simulink model "FOC_Motor_Tuning"  (R2025b)
settings: Solver=VariableStepAuto  StartTime=0.0  StopTime=8  RelTol=1e-3
values from neighbouring files (symbols this model uses):
  adc : value not decoded    [FoCFpgaData.sldd]
  dataRange = 800.0    [FoCFpgaData.sldd]
  encoder = 0.0    [FoCFpgaData.sldd]
  inverter = 24.0    [FoCFpgaData.sldd]
  paramAdcAmperePerCount : value not decoded    [FoCFpgaData.sldd]
  paramAdcCalibrationSamples = 16.0    [FoCFpgaData.sldd]
  paramAdcCountAtZeroAmpere : value not decoded    [FoCFpgaData.sldd]
  paramAdcEnablecalibration = 1.0    [FoCFpgaData.sldd]
  paramCurrentControlSatVoltage = 13.856406460551021    [FoCFpgaData.sldd]
  paramEncoderCalibrationDuration = 0.2    [FoCFpgaData.sldd]
  paramEncoderCalibrationMaxError = 0.0012566370614359172    [FoCFpgaData.sldd]
  paramEncoderCalibrationVoltage = 2.0    [FoCFpgaData.sldd]
  paramEncoderRotorPositionAtZeroCount = 0.0    [FoCFpgaData.sldd]
  paramOpenLoopVelocityAcceleration = 40.0    [FoCFpgaData.sldd]
  paramOpenLoopVelocityToVoltsBias = 0.4    [FoCFpgaData.sldd]
  paramOpenLoopVelocityToVoltsScalar = 0.04    [FoCFpgaData.sldd]
  paramOverCurrentDuration = 0.05    [FoCFpgaData.sldd]
  paramOverCurrentEnable = 0.0    [FoCFpgaData.sldd]
  paramOverCurrentLimit = 10.45    [FoCFpgaData.sldd]
  paramPwmCompareAtZeroVolt = 500.0    [FoCFpgaData.sldd]
  paramPwmCompareMax = 1000.0    [FoCFpgaData.sldd]
  paramPwmComparePerVolt = 41.666666666666664    [FoCFpgaData.sldd]
  paramVelocityControlSatCurrent = 3.5    [FoCFpgaData.sldd]
  PI_params = 0.00048000000000000007    [FoCFpgaData.sldd]
  pmsm : value not decoded    [FoCFpgaData.sldd]
  pwm = 2.0E-8    [FoCFpgaData.sldd]
  sampleTime = 4.0E-5    [FoCFpgaData.sldd]
libraries: fl_lib x12, nesl_utility x12, mcbeeMathTransformLib x8, simulink x4, slpidlib x4, ee_lib x4, mcbpositiondecoderlib x3, mcbcontrolslib x3, mcbplantlib x1, autolibpmsmexterior x1, eeGeneralControl x1, SignalEditorBlockLib x1
(part 3 of 3)

== system FOC_Motor_Tuning/FOC Control/Controller_Algorithm_Local/Algorithm_С/Open_Loop_Velocity_Control/Open_Loop_Velocity_Control/Inverse_Park_Transform ==
  note: Inverse Park Transform
  note: Converts orthogonal rotating reference frame (dq) to two-phase orthogonal stationary reference frame (alpha, beta)
  D : Inport
  Q : Inport  Port=2
  Sin_Coefficient : Inport  Port=3
  Cos_Coefficient : Inport  Port=4
  Add1 : Sum  Inputs=+-  OutDataTypeStr=Inherit: Same as first input
  Add2 : Sum  OutDataTypeStr=Inherit: Same as first input
  Cos_Coefficient1 : InportShadow  Port=4
  Product{1..4} (4 alike) : Product  RndMeth=Simplest
  Sin_Coefficient1 : InportShadow  Port=3
  Alpha : Outport  VectorParamsAs1DForOutWhenUnconnected=off
  Beta : Outport  Port=2  VectorParamsAs1DForOutWhenUnconnected=off
  wires:
  Add2/1 -> Beta/1
  Add1/1 -> Alpha/1
  Product3/1 -> Add2/1
  Product4/1 -> Add2/2
  Product1/1 -> Add1/1
  Product2/1 -> Add1/2
  Cos_Coefficient1/1 -> Product4/2
  Sin_Coefficient/1 -> Product2/2
  D/1 -> Product3/1, Product1/1
  Q/1 -> Product2/1, Product4/1
  Sin_Coefficient1/1 -> Product3/2
  Cos_Coefficient/1 -> Product1/2

== system FOC_Motor_Tuning/FOC Control/Controller_Algorithm_Local/Algorithm_С/Open_Loop_Velocity_Control/Open_Loop_Velocity_Control/Ramp_Velocity ==
  note: Ramp Velocity
  Velocity_Command : Inport
  Delay : Delay  DelayLength=1
  Gain : Gain  Gain=sampleTime.OpenLoopVelocityControl
      settings: AttributesFormatString=------------------------------\nGain = %<Gain>
  Number_Of_Pole_Pairs : Gain  Gain=pmsm.p
      settings: AttributesFormatString=------------------------------------\nGain = %<Gain>
  Set_Acceleration : Subsystem
  Sum : Sum  Inputs=++|  SaturateOnIntegerOverflow=on
  Rotor_Velocity : Outport  VectorParamsAs1DForOutWhenUnconnected=off
  Electrical_Velocity : Outport  Port=2  VectorParamsAs1DForOutWhenUnconnected=off
  wires:
  Number_Of_Pole_Pairs/1 -> Electrical_Velocity/1
  Set_Acceleration/1(A) -> Gain/1
  Velocity_Command/1 -> Set_Acceleration/1(V_Target)
  Gain/1 -> Sum/1
  Delay/1 -> Set_Acceleration/2(V_Current), Sum/2, Number_Of_Pole_Pairs/1, Rotor_Velocity/1
  Sum/1 -> Delay/1

== system FOC_Motor_Tuning/FOC Control/Controller_Algorithm_Local/Algorithm_С/Open_Loop_Velocity_Control/Open_Loop_Velocity_Control/Rotor_Velocity_To_Volts ==
  note: Rotor Velocity To Volts
  RV : Inport
  Abs : Abs  SaturateOnIntegerOverflow=off
  Add : Sum  OutDataTypeStr=Inherit: Same as first input
  Frequency_To_Voltage : Gain  Gain=paramOpenLoopVelocityToVoltsScalar
      settings: AttributesFormatString=--------------------------------\n%<Gain>
  Voltage_Bias : Constant  Value=paramOpenLoopVelocityToVoltsBias  OutDataTypeStr=Inherit: Inherit via back propagation  SampleTime=-1
  V : Outport  VectorParamsAs1DForOutWhenUnconnected=off
  wires:
  RV/1 -> Abs/1
  Abs/1 -> Frequency_To_Voltage/1
  Frequency_To_Voltage/1 -> Add/2
  Add/1 -> V/1
  Voltage_Bias/1 -> Add/1

== system FOC_Motor_Tuning/FOC Control/Controller_Algorithm_Local/Algorithm_HDL/FOC_Velocity_Encoder/FOC_Current_Control/FOC_Current_Control_Fixdt/DQ_Current_Control ==
  note: DQ Current Control
  Reset : Inport
  Q_Command : Inport  Port=2  SampleTime=sampleTime.CurrentControl
  D_Current : Inport  Port=3
  Q_Current : Inport  Port=4
  D_Command : Constant  Value=0  OutDataTypeStr=fixdt(1,16,0)  SampleTime=-1
  D_Control : slpidlib/PID Controller  Controller=PI  Form=Parallel  TimeDomain=Discrete-time  UseExternalTs=off  SampleTime=-1  IntegratorMethod=Forward Euler  FilterMethod=Forward Euler  ControllerParametersSource=external  P=1  I=1  UseKiTs=on  D=0  UseExternalDerivativeSource=off  N=100  UseFilter=on  TunerSelectOption=Transfer Function Based (PID Tuner App)  InitialConditionSource=internal  InitialConditionForIntegrator=0  InitialConditionForFilter=0  DifferentiatorICPrevScaledInput=0  ExternalReset=level  TrackingMode=off  Kt=1  LimitOutput=on  SatLimitsSource=internal  UpperSaturationLimit=paramCurrentControlSatVoltage  LowerSaturationLimit=-paramCurrentControlSatVoltage  LinearizeAsGain=on  AntiWindupMode=clamping  Kb=1  LimitIntegrator=off  UpperIntegratorSaturationLimit=inf  LowerIntegratorSaturationLimit=-inf  RndMeth=Simplest  POutMin=[]  POutMax=[]  IOutMin=[]  IOutMax=[]  DOutMin=[]  DOutMax=[]  NOutMin=[]  NOutMax=[]  SumOutMin=[]  SumOutMax=[]  SaturationOutDataTypeStr=Inherit: Inherit via back propagation  SaturationOutMin=[]  SaturationOutMax=[]  PParamMin=[]  PParamMax=[]  IParamMin=[]  IParamMax=[]  DParamMin=[]  DParamMax=[]  NParamMin=[]  NParamMax=[]  KbParamMin=[]  KbParamMax=[]  KtParamMin=[]  KtParamMax=[]  KbOutMin=[]  KbOutMax=[]  KtOutMin=[]  KtOutMax=[]  IntegratorOutMin=[]  IntegratorOutMax=[]  FilterOutMin=[]  FilterOutMax=[]  SumI1OutMin=[]  SumI1OutMax=[]  SumI2OutMin=[]  SumI2OutMax=[]  SumI3OutMin=[]  SumI3OutMax=[]  SumI4OutMin=[]  SumI4OutMax=[]  SumDOutMin=[]  SumDOutMax=[]  DifferentiatorOutMin=[]  DifferentiatorOutMax=[]  FilterDiffOutCoefMin=[]  FilterDiffOutCoefMax=[]  ReciprocalOutMin=[]  ReciprocalOutMax=[]  SumDenOutMin=[]  SumDenOutMax=[]  SumNumOutMin=[]  SumNumOutMax=[]  DivideOutMin=[]  DivideOutMax=[]  UdiffTsProdOutMin=[]  UdiffTsProdOutMax=[]  NTsProdOutMin=[]  NTsProdOutMax=[]  UintegralTsProdOutMin=[]  UintegralTsProdOutMax=[]  UngainTsProdOutMin=[]  UngainTsProdOutMax=[]  ClampingZeroOutDataTypeStr=Inherit: Inherit via back propagation  ClampingZeroOutMin=[]  ClampingZeroOutMax=[]  FilterDenConstantOutDataTypeStr=Inherit: Inherit via back propagation  FilterDenConstantOutMin=[]  FilterDenConstantOutMax=[]  PCopyOutDataTypeStr=Inherit: Inherit via back propagation  PCopyOutMin=[]  PCopyOutMax=[]  NCopyOutDataTypeStr=Inherit: Inherit via back propagation  NCopyOutMin=[]  NCopyOutMax=[]  IntegratorContinuousStateAttributes=''  IntegratorStateMustResolveToSignalObject=off  IntegratorRTWStateStorageClass=Auto  FilterContinuousStateAttributes=''  FilterStateMustResolveToSignalObject=off  FilterRTWStateStorageClass=Auto  ParallelPVariant=ExternalParameters  IdealPVariant=Disabled  IVariant=ExternalParameters  DVariant=Disabled  IntegratorVariant=Discrete  SatVariant=Enabled  AWVariant=DiscClampingParallel  PCopyVariant=Disabled  TRVariant=Disabled  FdbkBlocksVariant=Forward  IdealPFdbkVariant=Disabled  SatFdbkVariant=Disabled  DerivativeFilterVariant=Disabled  NVariant=Disabled  NCopyVariant=Disabled_SignalSpec  FilterICVariant=Disabled  IntegratorICVariant=InternalICs  ExternalResetVariant=ExternalReset  TRSumVariant=Passthrough  SumFdbkVariant=Disabled  SumVariant=Sum_PI  TsampFilterVariant=InternalTs  TsampNgainVariant=Passthrough  TsampIntegralVariant=Disabled_SignalSpec  ExternalSaturationOutDataTypeStr=Inherit: Same as second input  DerivativeSourceVariant=Disabled  PreIntVariant=InternalPreInt
      settings: LibrarySourceBlock=mcblib/Controls/Controllers/PI Controller
  Data_Type_Convert : DataTypeConversion  OutDataTypeStr=fixdt(1,16,11)  RndMeth=Simplest  SaturateOnIntegerOverflow=off
  Data_Type_Convert1 : DataTypeConversion  OutDataTypeStr=fixdt(1,16,11)  RndMeth=Simplest  SaturateOnIntegerOverflow=off
  Error : Sum  Inputs=+-  OutDataTypeStr=fixdt(1,32,24)
  Error1 : Sum  Inputs=+-  OutDataTypeStr=fixdt(1,32,24)
  Integral_Gain : Constant  Value=PI_params.Ki_i  OutDataTypeStr=fixdt(1,16,3)  SampleTime=-1
  Integral_Gain1 : Constant  Value=PI_params.Kp_i  OutDataTypeStr=fixdt(1,16,3)  SampleTime=-1
  Product : Product  OutDataTypeStr=fixdt(1,16,15)
  Q_Control : slpidlib/PID Controller  Controller=PI  Form=Parallel  TimeDomain=Discrete-time  UseExternalTs=off  SampleTime=-1  IntegratorMethod=Forward Euler  FilterMethod=Forward Euler  ControllerParametersSource=external  P=1  I=1  UseKiTs=on  D=0  UseExternalDerivativeSource=off  N=100  UseFilter=on  TunerSelectOption=Transfer Function Based (PID Tuner App)  InitialConditionSource=internal  InitialConditionForIntegrator=0  InitialConditionForFilter=0  DifferentiatorICPrevScaledInput=0  ExternalReset=level  TrackingMode=off  Kt=1  LimitOutput=on  SatLimitsSource=internal  UpperSaturationLimit=paramCurrentControlSatVoltage  LowerSaturationLimit=-paramCurrentControlSatVoltage  LinearizeAsGain=on  AntiWindupMode=clamping  Kb=1  LimitIntegrator=off  UpperIntegratorSaturationLimit=inf  LowerIntegratorSaturationLimit=-inf  RndMeth=Simplest  POutMin=[]  POutMax=[]  IOutMin=[]  IOutMax=[]  DOutMin=[]  DOutMax=[]  NOutMin=[]  NOutMax=[]  SumOutMin=[]  SumOutMax=[]  SaturationOutDataTypeStr=Inherit: Inherit via back propagation  SaturationOutMin=[]  SaturationOutMax=[]  PParamMin=[]  PParamMax=[]  IParamMin=[]  IParamMax=[]  DParamMin=[]  DParamMax=[]  NParamMin=[]  NParamMax=[]  KbParamMin=[]  KbParamMax=[]  KtParamMin=[]  KtParamMax=[]  KbOutMin=[]  KbOutMax=[]  KtOutMin=[]  KtOutMax=[]  IntegratorOutMin=[]  IntegratorOutMax=[]  FilterOutMin=[]  FilterOutMax=[]  SumI1OutMin=[]  SumI1OutMax=[]  SumI2OutMin=[]  SumI2OutMax=[]  SumI3OutMin=[]  SumI3OutMax=[]  SumI4OutMin=[]  SumI4OutMax=[]  SumDOutMin=[]  SumDOutMax=[]  DifferentiatorOutMin=[]  DifferentiatorOutMax=[]  FilterDiffOutCoefMin=[]  FilterDiffOutCoefMax=[]  ReciprocalOutMin=[]  ReciprocalOutMax=[]  SumDenOutMin=[]  SumDenOutMax=[]  SumNumOutMin=[]  SumNumOutMax=[]  DivideOutMin=[]  DivideOutMax=[]  UdiffTsProdOutMin=[]  UdiffTsProdOutMax=[]  NTsProdOutMin=[]  NTsProdOutMax=[]  UintegralTsProdOutMin=[]  UintegralTsProdOutMax=[]  UngainTsProdOutMin=[]  UngainTsProdOutMax=[]  ClampingZeroOutDataTypeStr=Inherit: Inherit via back propagation  ClampingZeroOutMin=[]  ClampingZeroOutMax=[]  FilterDenConstantOutDataTypeStr=Inherit: Inherit via back propagation  FilterDenConstantOutMin=[]  FilterDenConstantOutMax=[]  PCopyOutDataTypeStr=Inherit: Inherit via back propagation  PCopyOutMin=[]  PCopyOutMax=[]  NCopyOutDataTypeStr=Inherit: Inherit via back propagation  NCopyOutMin=[]  NCopyOutMax=[]  IntegratorContinuousStateAttributes=''  IntegratorStateMustResolveToSignalObject=off  IntegratorRTWStateStorageClass=Auto  FilterContinuousStateAttributes=''  FilterStateMustResolveToSignalObject=off  FilterRTWStateStorageClass=Auto  ParallelPVariant=ExternalParameters  IdealPVariant=Disabled  IVariant=ExternalParameters  DVariant=Disabled  IntegratorVariant=Discrete  SatVariant=Enabled  AWVariant=DiscClampingParallel  PCopyVariant=Disabled  TRVariant=Disabled  FdbkBlocksVariant=Forward  IdealPFdbkVariant=Disabled  SatFdbkVariant=Disabled  DerivativeFilterVariant=Disabled  NVariant=Disabled  NCopyVariant=Disabled_SignalSpec  FilterICVariant=Disabled  IntegratorICVariant=InternalICs  ExternalResetVariant=ExternalReset  TRSumVariant=Passthrough  SumFdbkVariant=Disabled  SumVariant=Sum_PI  TsampFilterVariant=InternalTs  TsampNgainVariant=Passthrough  TsampIntegralVariant=Disabled_SignalSpec  ExternalSaturationOutDataTypeStr=Inherit: Same as second input  DerivativeSourceVariant=Disabled  PreIntVariant=InternalPreInt
      settings: LibrarySourceBlock=mcblib/Controls/Controllers/PI Controller
  Reset1 : InportShadow
  Sample_Time : Constant  Value=sampleTime.CurrentControl  OutDataTypeStr=fixdt(1,16,27)  SampleTime=-1
  D_Voltage : Outport  VectorParamsAs1DForOutWhenUnconnected=off
  Q_Voltage : Outport  Port=2  VectorParamsAs1DForOutWhenUnconnected=off
  wires:
  Data_Type_Convert1/1 -> Q_Voltage/1
  D_Control/1 -> Data_Type_Convert/1
  D_Command/1 -> Error/1  "Id_Ref"
  Q_Command/1 -> Error1/1  "Iq_Ref"
  Q_Current/1 -> Error1/2  "Iq_Fb"
  D_Current/1 -> Error/2  "Id_Fb"
  Reset/1 -> D_Control/4
  Reset1/1 -> Q_Control/4
  Error/1 -> D_Control/1  "currentControlError"
  Product/1 -> Q_Control/3, D_Control/3
  Sample_Time/1 -> Product/2
  Integral_Gain/1 -> Product/1
  Integral_Gain1/1 -> Q_Control/2, D_Control/2
  Data_Type_Convert/1 -> D_Voltage/1
  Q_Control/1 -> Data_Type_Convert1/1
  Error1/1 -> Q_Control/1  "currentControlError"

== system FOC_Motor_Tuning/FOC Control/Controller_Algorithm_Local/Algorithm_HDL/FOC_Velocity_Encoder/FOC_Current_Control/FOC_Current_Control_Fixdt/Sine_Cosine ==
  note: Sine Cosine Fixed Point LUT
  P : Inport
  Normalize_Position : Gain  Gain=1/(2*pi)  ParamDataTypeStr=fixdt(1,16,17)  OutMin=0  OutMax=1  OutDataTypeStr=fixdt(1,32,30)
      settings: AttributesFormatString=|
      | ------------------------------
      | Gain = %<Gain>
  Sine_Cosine_LUT : simulink/Lookup Tables/Sine  Formula=sin(2*pi*u) and cos(2*pi*u)  NumDataPoints=(2^5)+1  OutputWordLength=16  InternalRulePriority=Speed
  Sin : Outport  VectorParamsAs1DForOutWhenUnconnected=off
  Cos : Outport  Port=2  VectorParamsAs1DForOutWhenUnconnected=off
  wires:
  Sine_Cosine_LUT/2 -> Cos/1
  Sine_Cosine_LUT/1 -> Sin/1
  Normalize_Position/1 -> Sine_Cosine_LUT/1
  P/1 -> Normalize_Position/1  "position"

== system FOC_Motor_Tuning/FOC Control/Controller_Algorithm_Local/Algorithm_HDL/FOC_Velocity_Encoder/FOC_Current_Control/FOC_Current_Control_Single/FOC_Current_Control ==
  note: FOC Current Control
  Reset : Inport  SampleTime=sampleTime.CurrentControl
  Current_Command : Inport  Port=2  OutMin=dataRange.PhaseCurrent.Min  OutMax=dataRange.PhaseCurrent.Max  SampleTime=sampleTime.CurrentControl
  Phase_Current : Inport  Port=3  OutMin=dataRange.PhaseCurrent.Min  OutMax=dataRange.PhaseCurrent.Max  SampleTime=sampleTime.CurrentControl
  Electrical_Position : Inport  Port=4  OutMin=0  OutMax=2*pi  SampleTime=sampleTime.CurrentControl
  Clarke Transform : mcbeeMathTransformLib/Clarke Transform  VariantControl=Variant2  PowerInvariant=off  UseWithEmbedded=on  PhaseInput=Two inputs
      settings: LibrarySourceBlock=mcbcontrolslib/Clarke Transform
  DQ_Current_Control : Subsystem
  Demux : Demux  Outputs=2
  Inverse Clarke Transform : mcbeeMathTransformLib/Inverse Clarke Transform  PowerInvariant=off  UseWithEmbedded=on  PhaseInput=Two inputs
      settings: LibrarySourceBlock=mcbcontrolslib/Inverse Clarke Transform
  Inverse Park Transform : mcbeeMathTransformLib/Park to Clarke Angle Transform  AxisAlignment=D-axis  UseWithEmbedded=on  PhaseInput=Two inputs  ThetaInput=Sine and Cosine electrical position  AngleInput=Per-unit  N_points=1024
      settings: LibrarySourceBlock=mcbcontrolslib/Inverse Park Transform
  Mux : Mux  Inputs=3
  PWM Reference Generator : mcbcontrolslib/PWM Reference Generator  inSignal=Vabc  modType=SVM: space vector modulation
      settings: LibrarySourceBlock=mcbhdllib/Controls/Math Transforms/PWM Reference Generator
  Park Transform : mcbeeMathTransformLib/Clarke to Park Angle Transform  AxisAlignment=D-axis  UseWithEmbedded=on  PhaseInput=Two inputs  ThetaInput=Sine and Cosine electrical position  AngleInput=Per-unit  N_points=1024
      settings: LibrarySourceBlock=mcbcontrolslib/Park Transform
  Sat : Saturate  UpperLimit=dataRange.PhaseVoltage.Max  LowerLimit=dataRange.PhaseVoltage.Min  OutDataTypeStr=Inherit: Inherit via back propagation
      settings: AttributesFormatString=-----------------\nLower = %<LowerLimit>\nUpper = %<UpperLimit>
  Trigonometric Function : Trigonometry  Operator=sincos
  Phase_Voltage : Outport  SampleTime=sampleTime.CurrentControl  VectorParamsAs1DForOutWhenUnconnected=off
  wires:
  Trigonometric Function/1 -> Inverse Park Transform/3, Park Transform/3  "sinCoefficient"
  Trigonometric Function/2 -> Inverse Park Transform/4, Park Transform/4  "cosCoefficient"
  Electrical_Position/1 -> Trigonometric Function/1
  Clarke Transform/1 -> Park Transform/1  "alphaCurrent"
  Clarke Transform/2 -> Park Transform/2  "betaCurrent"
  Inverse Park Transform/1 -> Inverse Clarke Transform/1  "alphaVoltage"
  Inverse Park Transform/2 -> Inverse Clarke Transform/2  "betaVoltage"
  Park Transform/1 -> DQ_Current_Control/3(D_Current)  "dCurrent"
  Park Transform/2 -> DQ_Current_Control/4(Q_Current)  "qCurrent"
  Current_Command/1 -> DQ_Current_Control/2(Q_Command)
  DQ_Current_Control/1(D_Voltage) -> Inverse Park Transform/1  "dVoltage"
  DQ_Current_Control/2(Q_Voltage) -> Inverse Park Transform/2  "qVoltage"
  Mux/1 -> Sat/1  "svmVoltage"
  Sat/1 -> Phase_Voltage/1
  Reset/1 -> DQ_Current_Control/1(Reset)
  Phase_Current/1 -> Demux/1
  Demux/1 -> Clarke Transform/1
  Demux/2 -> Clarke Transform/2
  Inverse Clarke Transform/1 -> PWM Reference Generator/1
  Inverse Clarke Transform/2 -> PWM Reference Generator/2
  Inverse Clarke Transform/3 -> PWM Reference Generator/3
  PWM Reference Generator/1 -> Mux/1
  PWM Reference Generator/2 -> Mux/2
  PWM Reference Generator/3 -> Mux/3

== system FOC_Motor_Tuning/FOC Control/Controller_Algorithm_Local/Algorithm_С/Open_Loop_Velocity_Control/Open_Loop_Velocity_Control/Electrical_Velocity_To_Position/Mod_Two_Pi_Once ==
  note: Mod Two Pi Once
  X : Inport
  Add1 : Sum  Inputs=+-
  Add2 : Sum
  Greater_Than : RelationalOperator  OutDataTypeStr=boolean  InputSameDT=off
  Input_Range : SignalSpecification  OutMin=-4*pi  OutMax=4*pi
      settings: AttributesFormatString=|
      | -----------------------
      | Min = %<OutMin>
      | Max = %<OutMax>
  Less_Than : RelationalOperator  Operator=<  OutDataTypeStr=boolean  InputSameDT=off
  Output_Range : SignalSpecification  OutMin=0  OutMax=2*pi
      settings: AttributesFormatString=|
      | -----------------------
      | Min = %<OutMin>
      | Max = %<OutMax>
  Switch : Switch  Criteria=u2 ~= 0  SaturateOnIntegerOverflow=off
  Switch1 : Switch  Criteria=u2 ~= 0  SaturateOnIntegerOverflow=off
  Two_Pi : Constant  Value=2*pi  OutDataTypeStr=Inherit: Inherit via back propagation
  Two_Pi1 : Constant  Value=2*pi  OutDataTypeStr=Inherit: Inherit via back propagation
  Two_Pi2 : Constant  Value=2*pi  OutDataTypeStr=Inherit: Inherit via back propagation
  Zero : Constant  Value=0  OutDataTypeStr=Inherit: Inherit via back propagation
  Mod_X_Two_Pi : Outport  VectorParamsAs1DForOutWhenUnconnected=off
  wires:
  Input_Range/1 -> Switch1/3, Less_Than/1, Add2/1, Greater_Than/1, Add1/1
  Switch/1 -> Output_Range/1
  X/1 -> Input_Range/1
  Greater_Than/1 -> Switch/2
  Add1/1 -> Switch/1
  Two_Pi/1 -> Add1/2
  Two_Pi1/1 -> Greater_Than/2
  Switch1/1 -> Switch/3
  Less_Than/1 -> Switch1/2
  Add2/1 -> Switch1/1
  Two_Pi2/1 -> Add2/2
  Zero/1 -> Less_Than/2
  Output_Range/1 -> Mod_X_Two_Pi/1

== system FOC_Motor_Tuning/FOC Control/Controller_Algorithm_Local/Algorithm_С/Open_Loop_Velocity_Control/Open_Loop_Velocity_Control/Ramp_Velocity/Set_Acceleration ==
  note: Set Acceleration
  V_Target : Inport
  V_Current : Inport  Port=2
  AND_Neg : Logic  IconShape=distinctive  AllPortsSameDT=off  OutDataTypeStr=boolean
  AND_Pos : Logic  IconShape=distinctive  AllPortsSameDT=off  OutDataTypeStr=boolean
  Acceleration : Constant  Value=paramOpenLoopVelocityAcceleration  OutDataTypeStr=Inherit: Inherit via back propagation  SampleTime=-1
  Delay1 : Delay  DelayLength=1
  Detect_Change : Subsystem
  Greater_Than : RelationalOperator  Operator=>  OutDataTypeStr=boolean  InputSameDT=off
  Latch_Target : Switch  Criteria=u2 ~= 0  SaturateOnIntegerOverflow=off  InputSameDT=off
  NOT1 : Logic  Operator=NOT  IconShape=distinctive  AllPortsSameDT=off  OutDataTypeStr=boolean
  NOT2 : Logic  Operator=NOT  IconShape=distinctive  AllPortsSameDT=off  OutDataTypeStr=boolean
  OR : Logic  Operator=OR  IconShape=distinctive  AllPortsSameDT=off  OutDataTypeStr=boolean
  Switch_Dir : Switch  Criteria=u2 > Threshold  SaturateOnIntegerOverflow=off  InputSameDT=off
  Switch_Stop : Switch  Criteria=u2 ~= 0  SaturateOnIntegerOverflow=off  InputSameDT=off
  Unary_Minus : UnaryMinus
  V_Target1 : InportShadow
  Zero : Constant  Value=0  OutDataTypeStr=Inherit: Inherit via back propagation  SampleTime=-1
  A : Outport  VectorParamsAs1DForOutWhenUnconnected=off
  wires:
  Latch_Target/1 -> AND_Pos/2, NOT2/1, Switch_Dir/2, Delay1/1  "positiveDirection"
  Greater_Than/1 -> NOT1/1, Latch_Target/1, AND_Neg/1  "currentLessThanTarget"
  Delay1/1 -> Latch_Target/3
  V_Current/1 -> Greater_Than/2
  V_Target1/1 -> Greater_Than/1
  V_Target/1 -> Detect_Change/1(X)
  Detect_Change/1(Y) -> Latch_Target/2  "targetHasChanged"
  Unary_Minus/1 -> Switch_Dir/3
  Acceleration/1 -> Unary_Minus/1, Switch_Dir/1  "positiveAccleration"
  Switch_Stop/1 -> A/1
  Switch_Dir/1 -> Switch_Stop/3  "accleration"
  Zero/1 -> Switch_Stop/1
  NOT1/1 -> AND_Pos/1  "currentGreaterThanTarget"
  AND_Pos/1 -> OR/1  "stopPositiveAcceleration"
  OR/1 -> Switch_Stop/2  "stopAccelerating"
  NOT2/1 -> AND_Neg/2  "negativeDirection"
  AND_Neg/1 -> OR/2  "stopNegativeAcceleration"

== system FOC_Motor_Tuning/FOC Control/Controller_Algorithm_Local/Algorithm_HDL/FOC_Velocity_Encoder/FOC_Current_Control/FOC_Current_Control_Single/FOC_Current_Control/DQ_Current_Control ==
  note: DQ Current Control
  Reset : Inport
  Q_Command : Inport  Port=2  SampleTime=sampleTime.CurrentControl
  D_Current : Inport  Port=3
  Q_Current : Inport  Port=4
  D_Command : Constant  Value=0  OutDataTypeStr=Inherit: Inherit via back propagation  SampleTime=-1
  D_Control : slpidlib/PID Controller  Controller=PI  Form=Parallel  TimeDomain=Discrete-time  UseExternalTs=off  SampleTime=-1  IntegratorMethod=Forward Euler  FilterMethod=Forward Euler  ControllerParametersSource=external  P=1  I=1  UseKiTs=on  D=0  UseExternalDerivativeSource=off  N=100  UseFilter=on  TunerSelectOption=Transfer Function Based (PID Tuner App)  InitialConditionSource=internal  InitialConditionForIntegrator=0  InitialConditionForFilter=0  DifferentiatorICPrevScaledInput=0  ExternalReset=level  TrackingMode=off  Kt=1  LimitOutput=on  SatLimitsSource=internal  UpperSaturationLimit=paramCurrentControlSatVoltage  LowerSaturationLimit=-paramCurrentControlSatVoltage  LinearizeAsGain=on  AntiWindupMode=back-calculation  Kb=1  LimitIntegrator=off  UpperIntegratorSaturationLimit=inf  LowerIntegratorSaturationLimit=-inf  RndMeth=Simplest  POutMin=[]  POutMax=[]  IOutMin=[]  IOutMax=[]  DOutMin=[]  DOutMax=[]  NOutMin=[]  NOutMax=[]  SumOutMin=[]  SumOutMax=[]  SaturationOutDataTypeStr=Inherit: Inherit via back propagation  SaturationOutMin=[]  SaturationOutMax=[]  PParamMin=[]  PParamMax=[]  IParamMin=[]  IParamMax=[]  DParamMin=[]  DParamMax=[]  NParamMin=[]  NParamMax=[]  KbParamMin=[]  KbParamMax=[]  KtParamMin=[]  KtParamMax=[]  KbOutMin=[]  KbOutMax=[]  KtOutMin=[]  KtOutMax=[]  IntegratorOutMin=[]  IntegratorOutMax=[]  FilterOutMin=[]  FilterOutMax=[]  SumI1OutMin=[]  SumI1OutMax=[]  SumI2OutMin=[]  SumI2OutMax=[]  SumI3OutMin=[]  SumI3OutMax=[]  SumI4OutMin=[]  SumI4OutMax=[]  SumDOutMin=[]  SumDOutMax=[]  DifferentiatorOutMin=[]  DifferentiatorOutMax=[]  FilterDiffOutCoefMin=[]  FilterDiffOutCoefMax=[]  ReciprocalOutMin=[]  ReciprocalOutMax=[]  SumDenOutMin=[]  SumDenOutMax=[]  SumNumOutMin=[]  SumNumOutMax=[]  DivideOutMin=[]  DivideOutMax=[]  UdiffTsProdOutMin=[]  UdiffTsProdOutMax=[]  NTsProdOutMin=[]  NTsProdOutMax=[]  UintegralTsProdOutMin=[]  UintegralTsProdOutMax=[]  UngainTsProdOutMin=[]  UngainTsProdOutMax=[]  ClampingZeroOutDataTypeStr=Inherit: Inherit via back propagation  ClampingZeroOutMin=[]  ClampingZeroOutMax=[]  FilterDenConstantOutDataTypeStr=Inherit: Inherit via back propagation  FilterDenConstantOutMin=[]  FilterDenConstantOutMax=[]  PCopyOutDataTypeStr=Inherit: Inherit via back propagation  PCopyOutMin=[]  PCopyOutMax=[]  NCopyOutDataTypeStr=Inherit: Inherit via back propagation  NCopyOutMin=[]  NCopyOutMax=[]  IntegratorContinuousStateAttributes=''  IntegratorStateMustResolveToSignalObject=off  IntegratorRTWStateStorageClass=Auto  FilterContinuousStateAttributes=''  FilterStateMustResolveToSignalObject=off  FilterRTWStateStorageClass=Auto  ParallelPVariant=ExternalParameters  IdealPVariant=Disabled  IVariant=ExternalParameters  DVariant=Disabled  IntegratorVariant=Discrete  SatVariant=Enabled  AWVariant=BackCalculation  PCopyVariant=Disabled  TRVariant=Disabled  FdbkBlocksVariant=Forward  IdealPFdbkVariant=Disabled  SatFdbkVariant=Disabled  DerivativeFilterVariant=Disabled  NVariant=Disabled  NCopyVariant=Disabled_SignalSpec  FilterICVariant=Disabled  IntegratorICVariant=InternalICs  ExternalResetVariant=ExternalReset  TRSumVariant=Passthrough  SumFdbkVariant=Disabled  SumVariant=Sum_PI  TsampFilterVariant=InternalTs  TsampNgainVariant=Passthrough  TsampIntegralVariant=Disabled_SignalSpec  ExternalSaturationOutDataTypeStr=Inherit: Same as second input  DerivativeSourceVariant=Disabled  PreIntVariant=InternalPreInt
      settings: LibrarySourceBlock=mcblib/Controls/Controllers/PI Controller
  Error : Sum  Inputs=+-  OutDataTypeStr=single
  Error1 : Sum  Inputs=+-  OutDataTypeStr=single
  Integral_Gain : Constant  Value=PI_params.Ki_i  OutDataTypeStr=single  SampleTime=-1
  Integral_Gain1 : Constant  Value=PI_params.Kp_i  OutDataTypeStr=single  SampleTime=-1
  Product : Product  OutDataTypeStr=single
  Q_Control : slpidlib/PID Controller  Controller=PI  Form=Parallel  TimeDomain=Discrete-time  UseExternalTs=off  SampleTime=-1  IntegratorMethod=Forward Euler  FilterMethod=Forward Euler  ControllerParametersSource=external  P=1  I=1  UseKiTs=on  D=0  UseExternalDerivativeSource=off  N=100  UseFilter=on  TunerSelectOption=Transfer Function Based (PID Tuner App)  InitialConditionSource=internal  InitialConditionForIntegrator=0  InitialConditionForFilter=0  DifferentiatorICPrevScaledInput=0  ExternalReset=level  TrackingMode=off  Kt=1  LimitOutput=on  SatLimitsSource=internal  UpperSaturationLimit=paramCurrentControlSatVoltage  LowerSaturationLimit=-paramCurrentControlSatVoltage  LinearizeAsGain=on  AntiWindupMode=back-calculation  Kb=1  LimitIntegrator=off  UpperIntegratorSaturationLimit=inf  LowerIntegratorSaturationLimit=-inf  RndMeth=Simplest  POutMin=[]  POutMax=[]  IOutMin=[]  IOutMax=[]  DOutMin=[]  DOutMax=[]  NOutMin=[]  NOutMax=[]  SumOutMin=[]  SumOutMax=[]  SaturationOutDataTypeStr=Inherit: Inherit via back propagation  SaturationOutMin=[]  SaturationOutMax=[]  PParamMin=[]  PParamMax=[]  IParamMin=[]  IParamMax=[]  DParamMin=[]  DParamMax=[]  NParamMin=[]  NParamMax=[]  KbParamMin=[]  KbParamMax=[]  KtParamMin=[]  KtParamMax=[]  KbOutMin=[]  KbOutMax=[]  KtOutMin=[]  KtOutMax=[]  IntegratorOutMin=[]  IntegratorOutMax=[]  FilterOutMin=[]  FilterOutMax=[]  SumI1OutMin=[]  SumI1OutMax=[]  SumI2OutMin=[]  SumI2OutMax=[]  SumI3OutMin=[]  SumI3OutMax=[]  SumI4OutMin=[]  SumI4OutMax=[]  SumDOutMin=[]  SumDOutMax=[]  DifferentiatorOutMin=[]  DifferentiatorOutMax=[]  FilterDiffOutCoefMin=[]  FilterDiffOutCoefMax=[]  ReciprocalOutMin=[]  ReciprocalOutMax=[]  SumDenOutMin=[]  SumDenOutMax=[]  SumNumOutMin=[]  SumNumOutMax=[]  DivideOutMin=[]  DivideOutMax=[]  UdiffTsProdOutMin=[]  UdiffTsProdOutMax=[]  NTsProdOutMin=[]  NTsProdOutMax=[]  UintegralTsProdOutMin=[]  UintegralTsProdOutMax=[]  UngainTsProdOutMin=[]  UngainTsProdOutMax=[]  ClampingZeroOutDataTypeStr=Inherit: Inherit via back propagation  ClampingZeroOutMin=[]  ClampingZeroOutMax=[]  FilterDenConstantOutDataTypeStr=Inherit: Inherit via back propagation  FilterDenConstantOutMin=[]  FilterDenConstantOutMax=[]  PCopyOutDataTypeStr=Inherit: Inherit via back propagation  PCopyOutMin=[]  PCopyOutMax=[]  NCopyOutDataTypeStr=Inherit: Inherit via back propagation  NCopyOutMin=[]  NCopyOutMax=[]  IntegratorContinuousStateAttributes=''  IntegratorStateMustResolveToSignalObject=off  IntegratorRTWStateStorageClass=Auto  FilterContinuousStateAttributes=''  FilterStateMustResolveToSignalObject=off  FilterRTWStateStorageClass=Auto  ParallelPVariant=ExternalParameters  IdealPVariant=Disabled  IVariant=ExternalParameters  DVariant=Disabled  IntegratorVariant=Discrete  SatVariant=Enabled  AWVariant=BackCalculation  PCopyVariant=Disabled  TRVariant=Disabled  FdbkBlocksVariant=Forward  IdealPFdbkVariant=Disabled  SatFdbkVariant=Disabled  DerivativeFilterVariant=Disabled  NVariant=Disabled  NCopyVariant=Disabled_SignalSpec  FilterICVariant=Disabled  IntegratorICVariant=InternalICs  ExternalResetVariant=ExternalReset  TRSumVariant=Passthrough  SumFdbkVariant=Disabled  SumVariant=Sum_PI  TsampFilterVariant=InternalTs  TsampNgainVariant=Passthrough  TsampIntegralVariant=Disabled_SignalSpec  ExternalSaturationOutDataTypeStr=Inherit: Same as second input  DerivativeSourceVariant=Disabled  PreIntVariant=InternalPreInt
      settings: LibrarySourceBlock=mcblib/Controls/Controllers/PI Controller
  Reset1 : InportShadow
  Sample_Time : Constant  Value=sampleTime.CurrentControl  OutDataTypeStr=single  SampleTime=-1
  D_Voltage : Outport  VectorParamsAs1DForOutWhenUnconnected=off
  Q_Voltage : Outport  Port=2  VectorParamsAs1DForOutWhenUnconnected=off
  wires:
  Q_Control/1 -> Q_Voltage/1
  D_Control/1 -> D_Voltage/1
  D_Command/1 -> Error/1  "Id_Ref"
  Q_Command/1 -> Error1/1  "Iq_Ref"
  Q_Current/1 -> Error1/2  "Iq_Fb"
  D_Current/1 -> Error/2  "Id_Fb"
  Reset/1 -> D_Control/4
  Reset1/1 -> Q_Control/4
  Error/1 -> D_Control/1  "currentControlError"
  Error1/1 -> Q_Control/1  "currentControlError"
  Integral_Gain1/1 -> Q_Control/2, D_Control/2
  Integral_Gain/1 -> Product/1
  Sample_Time/1 -> Product/2
  Product/1 -> Q_Control/3, D_Control/3

== system FOC_Motor_Tuning/FOC Control/Controller_Algorithm_Local/Algorithm_С/Open_Loop_Velocity_Control/Open_Loop_Velocity_Control/Ramp_Velocity/Set_Acceleration/Detect_Change ==
  note: Detect Change
  X : Inport
  Add : Sum  Inputs=+-
  Delay : Delay  DelayLength=1
  Not_Equal_Zero : simulink/Logic and Bit Operations/Compare To Zero  relop=~=  OutDataTypeStr=boolean
  Y : Outport  VectorParamsAs1DForOutWhenUnconnected=off
  wires:
  X/1 -> Delay/1, Add/1
  Not_Equal_Zero/1 -> Y/1
  Add/1 -> Not_Equal_Zero/1
  Delay/1 -> Add/2

== stateflow chart FOC_Motor_Tuning/FOC Control/Controller_Algorithm_Local/Algorithm_С/Mode_Scheduler ==
  settings: updateMethod=DISCRETE
  note: Mode Scheduler
  state Enable_Inverter
    state Open_Loop
      state Open_Loop_Command
      state Find_Encoder_Index
    state Calibrate_Encoder_Offset
    state Closed_Loop
    (junction 378) -> Open_Loop_Command [order 1] : [commandType == ...
        |  commandTypeEnum.OpenLoopVelocity]
    (junction 378) -> (junction 624) [order 2]
    Open_Loop_Command -> (junction 624) : [commandType ~= ...
        |  commandTypeEnum.OpenLoopVelocity]
    (junction 624) -> (junction 619)
    (junction 619) -> (junction 638) [order 1] : [(commandType == ...
        |   commandTypeEnum.CalibrateEncoder) ...
        |  || (paramEncoderCalibrateAtStartup ...
        |      && ~encoderOffsetFound) ]
    (junction 638) -> Find_Encoder_Index [order 1] : [~encoderIndexFound]
    (junction 638) -> (junction 640) [order 2]
    (junction 619) -> (junction 604) [order 2]
    Find_Encoder_Index -> Calibrate_Encoder_Offset : [encoderIndexFound]
    (junction 640) -> Calibrate_Encoder_Offset
    Calibrate_Encoder_Offset -> (junction 604) : [(commandType ~= ...
        |   commandTypeEnum.CalibrateEncoder) ...
        |   && encoderOffsetFound]
    (junction 604) -> (junction 232)
    (junction 232) -> Closed_Loop [order 1] : [commandType == ...
        |  commandTypeEnum.Velocity]
    (junction 232) -> (junction 627) [order 2]
    Closed_Loop -> (junction 627) : [commandType ~= ...
        |  commandTypeEnum.Velocity]
  state Stand_By
    entry:
    if ~adcCalibrationStatus
    adcCalibration = boolean(1);
    end
    exit:
    adcCalibration = boolean(0);
  state Error
  (default) -> Stand_By
  Stand_By -> (junction 378) : [motorOn && adcCalibrationStatus]
  Enable_Inverter -> Stand_By [order 1] : [~motorOn]
  Error -> Stand_By : [~motorOn]
  Enable_Inverter -> Error [order 2] : [error]
  (junction 627) -> Error
  data: mode output Enum: modeSchedulerEnum; enableInverter output boolean; motorOn input; commandType input; encoderIndexFound input; openLoop output boolean; calibrateEncoder output boolean; closedLoop output boolean; encoderOffsetFound input; error input; paramEncoderCalibrateAtStartup parameter boolean; adcCalibrationStatus input; adcCalibration output

== matlab function FOC_Motor_Tuning/FOC Control/Controller_Algorithm_Local/Algorithm_С/ADC_Calibration/MATLAB Function ==
  data: ADCCounts input; ADCOffsetPhA output; Samples input; ADCOffsetPhB output; Flag output; EnCalibration input; ADCOffsets input
function [ADCOffsetPhA, ADCOffsetPhB, Flag]  = fcn(ADCCounts, Samples, EnCalibration, ADCOffsets)

persistent count;
if isempty(count)
	count = single(0);
end

persistent accumulator1;
if isempty(accumulator1) 
	accumulator1 = single(0);
end

persistent accumulator2;
if isempty(accumulator2)
	accumulator2 = single(0);
end
persistent out1; % initalize to meaningful ADC Offset
if isempty(out1)
	out1 = single(ADCOffsets(1));
end
persistent out2;
if isempty(out2)
	out2 = single(ADCOffsets(2));
end
persistent out3;
if isempty(out3)
	out3 = boolean(0);
end

%%
if EnCalibration  % Run the calibration
    if count < Samples
        accumulator1 = accumulator1 + ADCCounts(1);
        accumulator2 = accumulator2 + ADCCounts(2);
        count = count +single(1);
    else
        out1 = single(accumulator1/count);
        out2 = single(accumulator2/count);
        out3 = boolean(1);
    end
    
    ADCOffsetPhA = out1;
    ADCOffsetPhB = out2;
    Flag  = out3; 
else % use the ADC offsets provided 
    ADCOffsetPhA = ADCOffsets(1);
    ADCOffsetPhB = ADCOffsets(2) ;
    Flag  = boolean(1);
end


end

== stateflow chart FOC_Motor_Tuning/FOC Control/Controller_Algorithm_Local/Algorithm_HDL/FOC_Velocity_Encoder/Over_Current_Detector/Detect_Over_Current_Error ==
  settings: executeAtInitialization=1
  note: Detect Over Current Error
  note: If either Phase A Current (current[0]) or Phase B Current are above the threshold for a given duration, generate an error.
      | The error is reset when over current detection is disabled.
  state No_Error
    entry: error = false;
  state Possible_Error
  state Wait_For_Reset
  state Error
    entry: error = true;
  (default) -> No_Error
  No_Error -> Possible_Error : [enableOverCurrentDetect && ...
      |  ((phaseCurrentA >= overCurrentLimit) || ...
      |   (phaseCurrentB >= overCurrentLimit)    ) ]
  Possible_Error -> No_Error [order 1] : [(phaseCurrentA < overCurrentLimit) && ...
      |  (phaseCurrentB< overCurrentLimit)]
  Wait_For_Reset -> No_Error : [enableOverCurrentDetect]
  Possible_Error -> Error [order 2] : [after(overCurrentDurationTicks,tick)]
  Error -> Wait_For_Reset : [~enableOverCurrentDetect]
  data: enableOverCurrentDetect input; phaseCurrentA input; phaseCurrentB input; overCurrentLimit input; overCurrentDurationTicks input; error output boolean
